simulink model "ss_inter_jointActuationOff_i"  (R2019a)
settings: Solver=ode14x  StartTime=beginTime  StopTime=0.456  FixedStep=1e-4  RelTol=1e-3  EnableMultiTasking=on
model workspace (MAT data in the model file):
  Ankle_L_D = 1.86999822456
  Ankle_L_S = 0.0237763920936
  Ankle_R_D = 0.0588397140494
  Ankle_R_S = 0.739584271752
  F_C = 0.0618
  F_H = 0.107
  F_I = 0.0129
  F_L = 0.2471
  F_M = 1.2499
  F_W = 0.11
  GRF_HD = 42097.5090581
  GRF_HS = 111995.804745
  GRF_VD = 23523.4518935
  GRF_VS = 88551.3661398
  HAT_I = 4.3688
  HAT_L = 0.549
  HAT_M = 58.9182
  HAT_a = 0.2
  HAT_b = 0.13
  Hip_L_D = 0.00120944164738
  Hip_L_S = 1.91959156409
  Hip_R_D = 0.00174333284727
  Hip_R_S = 0.483982271561
  Knee_L_D = 0.900041230997
  Knee_L_S = 0.0187606009115
  Knee_R_D = 0.0722123401531
  Knee_R_S = 0.0187606009115
  M : struct (value not decoded)
  S_I = 0.073
  S_L = 0.447
  S_M = 4.0083
  S_R1 = 0.06
  S_R2 = 0.08
  T_I = 0.2042
  T_L = 0.476
  T_M = 8.62
  T_R1 = 0.08
  T_R2 = 0.1
  beginTime = 0.3901
  bodymass = 86.2
  lagStanceAnkle = [0 0 0 0 0 0]
  lagSwingAnkle = [0 0 0 0 0 0]
  lagSwingHip = [0 0 0 0 0 0]
  lagSwingKnee = [0 0 0 0 0 0]
  p_stance_ankle_i = 3.55956197506
  p_stance_hip_i = 21.6004762383
  p_stance_knee_i = -12.8836273009
  p_swing_ankle_i = -27.383897683
  p_swing_hip_i = -13.5921199012
  p_swing_knee_i = -0.51732567049
  polyfit_stance_ankle = [7.25005766341 -2.94260084728 3.61751641686 -0.1600680665]
  polyfit_swing_ankle = [-11368.0037517 20285.4827832 -14825.218273 5697.61347658 -1221.0674564 140.988649334 -7.60353693637 0.110238664523]
  polyfit_swing_hip = [-6497.04836191 6353.1189755 -1512.41069047 -218.046365216 114.745718447 -9.14187395017 -0.14056630138]
  polyfit_swing_knee = [20801.7792641 -51031.8985583 53804.8965773 -29864.6420618 9069.83319333 -1458.09150169 107.955966741 -2.65469998779 0.0787369748099]
  w_stance_ankle_i = -1.06696204007
  w_stance_hip_i = -58.6985398896
  w_stance_knee_i = 45.4476699768
  w_swing_ankle_i = 309.084119742
  w_swing_hip_i = 154.186680775
  w_swing_knee_i = 4.5424934361
  x_planar_p_i = 1.57252896947e-05
  x_planar_v_i = 0.000279430424888
  y_planar_p_i = -0.000501872604964
  y_planar_v_i = -0.011425534704
  z_planar_p_i = -0.153887861473
  z_planar_v_i = -3.47902548118
values from neighbouring files (symbols this model uses):
  N = 3    [lagdmodel.m]
symbols that are objects in the model workspace (value not decoded): M
undefined symbols (not defined in the file or in its folder): X, Y, Z
libraries: nesl_utility x62, sm_lib x46, fl_lib x24, fl_ps_legacy_lib x14
(part 7 of 7)

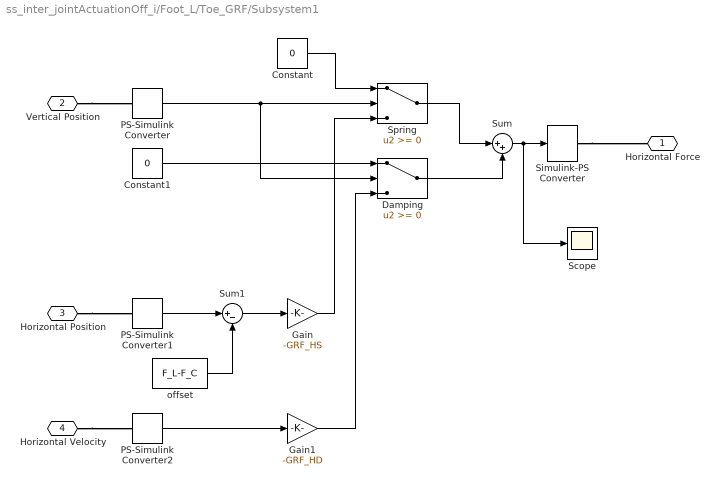
== system ss_inter_jointActuationOff_i/Foot_L/Toe_GRF/Subsystem1 ==
  Constant : Constant  Value=0
  Constant1 : Constant  Value=0
  Damping : Switch
  Gain : Gain  Gain=-GRF_HS
  Gain1 : Gain  Gain=-GRF_HD
  PS-Simulink Converter : nesl_utility/PS-Simulink Converter  PhysicalDomain=network_engine_domain  SubClassName=ps_output  LeftPortType=input  RightPortType=output  PseudoPeriodic=off  Frequencies=[]  Unit=1  AffineConversion=off
  PS-Simulink Converter1 : nesl_utility/PS-Simulink Converter  PhysicalDomain=network_engine_domain  SubClassName=ps_output  LeftPortType=input  RightPortType=output  PseudoPeriodic=off  Frequencies=[]  Unit=1  AffineConversion=off
  PS-Simulink Converter2 : nesl_utility/PS-Simulink Converter  PhysicalDomain=network_engine_domain  SubClassName=ps_output  LeftPortType=input  RightPortType=output  PseudoPeriodic=off  Frequencies=[]  Unit=1  AffineConversion=off
  Scope : Scope
  Simulink-PS Converter : nesl_utility/Simulink-PS Converter  PhysicalDomain=network_engine_domain  SubClassName=ps_input  LeftPortType=input  RightPortType=output  PseudoPeriodic=off  Frequencies=[]  NoiseDistribution=none  NoiseParameters=[]  Unit=1  AffineConversion=off  FilteringAndDerivatives=zero  SimscapeFilterOrder=1  InputFilterTimeConstant=.001  UdotUserProvided=[]
  Spring : Switch
  Sum : Sum  Inputs=|++
  Sum1 : Sum  Inputs=|+-
  "offset " : Constant  Value=F_L-F_C
  Horizontal Force : PMIOPort  Side=Right
  Vertical Position : PMIOPort  Port=2  Side=Left
  Horizontal Position : PMIOPort  Port=3  Side=Left
  Horizontal Velocity : PMIOPort  Port=4  Side=Left
  wires:
  PS-Simulink Converter/1 -> Spring/2, Damping/2
  Constant/1 -> Spring/1
  Sum/1 -> Scope/1, Simulink-PS Converter/1
  Spring/1 -> Sum/1
  Damping/1 -> Sum/2
  Constant1/1 -> Damping/1
  PS-Simulink Converter2/1 -> Gain1/1
  Gain/1 -> Spring/3
  Gain1/1 -> Damping/3
  PS-Simulink Converter1/1 -> Sum1/1
  "offset "/1 -> Sum1/2
  Sum1/1 -> Gain/1
  connections:
  Vertical Position/RConn1 -- PS-Simulink Converter/LConn1
  Horizontal Position/RConn1 -- PS-Simulink Converter1/LConn1
  Horizontal Velocity/RConn1 -- PS-Simulink Converter2/LConn1
  Simulink-PS Converter/RConn1 -- Horizontal Force/RConn1

== system ss_inter_jointActuationOff_i/Hip_L_Actuation/Hard_Stop_Hip_L/Rotational Simscape Intf (Library Block) ==
  Ideal Angular Velocity Source : fl_lib/Mechanical/Mechanical Sources/Ideal Angular Velocity Source
  Ideal Torque Sensor : fl_lib/Mechanical/Mechanical Sensors/Ideal Torque Sensor
  w : PMIOPort  Side=Left
  T : PMIOPort  Port=2  Side=Right
  R : PMIOPort  Port=3  Side=Left
  C : PMIOPort  Port=4  Side=Right
  connections:
  w/RConn1 -- Ideal Angular Velocity Source/RConn1
  T/RConn1 -- Ideal Torque Sensor/RConn2
  Ideal Torque Sensor/LConn1 -- Ideal Angular Velocity Source/RConn2
  R/RConn1 -- Ideal Angular Velocity Source/LConn1
  Ideal Torque Sensor/RConn1 -- C/RConn1

== system ss_inter_jointActuationOff_i/Hip_R_Actuation/Hard_Stop_Hip_R/Rotational Simscape Intf (Library Block) ==
  Ideal Angular Velocity Source : fl_lib/Mechanical/Mechanical Sources/Ideal Angular Velocity Source
  Ideal Torque Sensor : fl_lib/Mechanical/Mechanical Sensors/Ideal Torque Sensor
  w : PMIOPort  Side=Left
  T : PMIOPort  Port=2  Side=Right
  R : PMIOPort  Port=3  Side=Left
  C : PMIOPort  Port=4  Side=Right
  connections:
  w/RConn1 -- Ideal Angular Velocity Source/RConn1
  T/RConn1 -- Ideal Torque Sensor/RConn2
  Ideal Torque Sensor/LConn1 -- Ideal Angular Velocity Source/RConn2
  R/RConn1 -- Ideal Angular Velocity Source/LConn1
  Ideal Torque Sensor/RConn1 -- C/RConn1

== system ss_inter_jointActuationOff_i/Knee_L_Actuation/Hard_Stop_Knee_L/Rotational Simscape Intf (Library Block) ==
  Ideal Angular Velocity Source : fl_lib/Mechanical/Mechanical Sources/Ideal Angular Velocity Source
  Ideal Torque Sensor : fl_lib/Mechanical/Mechanical Sensors/Ideal Torque Sensor
  w : PMIOPort  Side=Left
  T : PMIOPort  Port=2  Side=Right
  R : PMIOPort  Port=3  Side=Left
  C : PMIOPort  Port=4  Side=Right
  connections:
  Ideal Torque Sensor/RConn1 -- C/RConn1
  R/RConn1 -- Ideal Angular Velocity Source/LConn1
  Ideal Torque Sensor/LConn1 -- Ideal Angular Velocity Source/RConn2
  T/RConn1 -- Ideal Torque Sensor/RConn2
  w/RConn1 -- Ideal Angular Velocity Source/RConn1

== system ss_inter_jointActuationOff_i/Knee_R_Actuation/Hard_Stop_Knee_L1/Rotational Simscape Intf (Library Block) ==
  Ideal Angular Velocity Source : fl_lib/Mechanical/Mechanical Sources/Ideal Angular Velocity Source
  Ideal Torque Sensor : fl_lib/Mechanical/Mechanical Sensors/Ideal Torque Sensor
  w : PMIOPort  Side=Left
  T : PMIOPort  Port=2  Side=Right
  R : PMIOPort  Port=3  Side=Left
  C : PMIOPort  Port=4  Side=Right
  connections:
  Ideal Torque Sensor/RConn1 -- C/RConn1
  R/RConn1 -- Ideal Angular Velocity Source/LConn1
  Ideal Torque Sensor/LConn1 -- Ideal Angular Velocity Source/RConn2
  T/RConn1 -- Ideal Torque Sensor/RConn2
  w/RConn1 -- Ideal Angular Velocity Source/RConn1
